simulink model "SchemaBlocFinala"  (R2024b)
settings: Solver=VariableStepAuto  StartTime=0.0  StopTime=1000  RelTol=1e-3
values from neighbouring files (symbols this model uses):
  A = 332.5    [date_indrumator.m]
  C = 9    [date_indrumator.m]
  h0 = 10.5    [date_indrumator.m]
  k = 0.035    [date_indrumator.m]    (also in proiect.m)
  k11 = k2^2 + 4*(k - k3)*k1    (= 0.08909684)    [date_indrumator.m]    (also in proiect.m = 0.08885985)
  k12 = 8*(k-k3)    (= 0.2848)    [date_indrumator.m]    (also in proiect.m)
  k13 = 2*(k-k3)    (= 0.0712)    [date_indrumator.m]    (also in proiect.m)
  k2 = -0.015    [date_indrumator.m]    (also in proiect.m = -0.0015)
  keta = 8*(10^-5)    (= 8e-05)    [date_indrumator.m]    (also in proiect.m)
  q0 = 29.18    [date_indrumator.m]
settings Model: Creator=Ruxandra  LastModifiedBy=Ruxandra

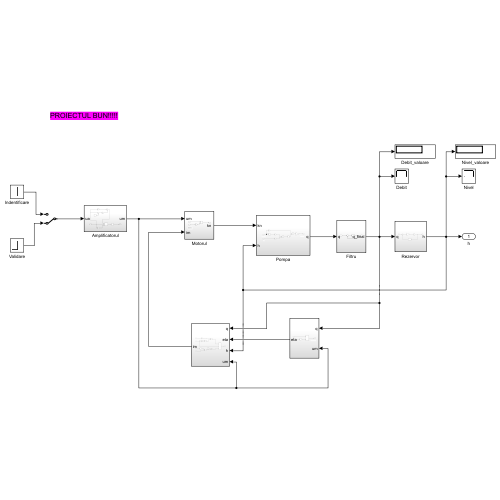
[thumbnail: Simulink's stored preview of the top-level diagram]
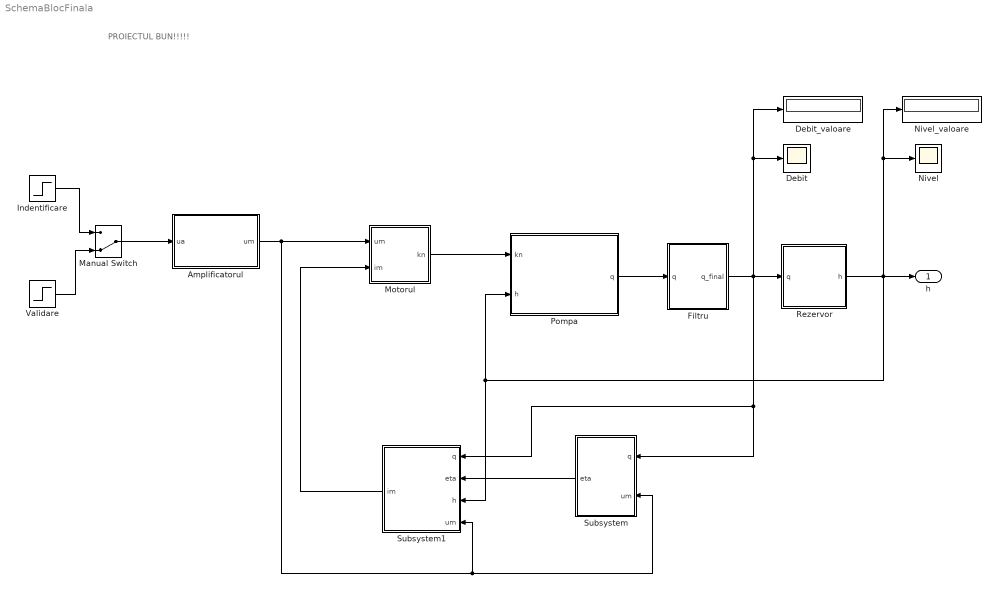
== system SchemaBlocFinala ==
  note: PROIECTUL BUN!!!!!
  Amplificatorul : Subsystem
  Debit : Scope
  Debit_valoare : Display
  Filtru : Subsystem
  Indentificare : Step  After=5  SampleTime=0
  Manual Switch : ManualSwitch  CurrentSetting=0
  Motorul : Subsystem
  Nivel : Scope
  Nivel_valoare : Display
  Pompa : Subsystem
  Rezervor : Subsystem
  Subsystem : Subsystem
  Subsystem1 : Subsystem
  Validare : Step  Before=5  After=5.5  SampleTime=0
  h : Outport
  wires:
  Motorul/1("kn ") -> Pompa/1(kn)
  Subsystem/1(eta) -> Subsystem1/2(eta)
  Subsystem1/1(im) -> Motorul/2(im)
  Pompa/1(q) -> Filtru/1(q)
  Filtru/1(q_final) -> Debit_valoare/1, Debit/1, Subsystem1/1(q), Subsystem/1(q), Rezervor/1(q)
  Rezervor/1(h) -> Pompa/2(h), Subsystem1/3(h), Nivel_valoare/1, Nivel/1, h/1
  Amplificatorul/1(um) -> Motorul/1(um), Subsystem1/4(um), Subsystem/2(um)
  Manual Switch/1 -> Amplificatorul/1(ua)
  Indentificare/1 -> Manual Switch/1
  Validare/1 -> Manual Switch/2

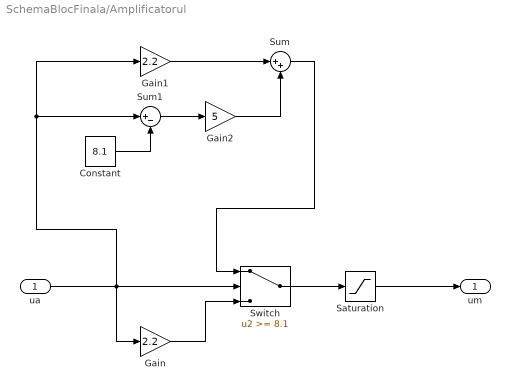
== system SchemaBlocFinala/Amplificatorul ==
  ua : Inport
  Constant : Constant  Value=8.1
  Gain : Gain  Gain=2.2
  Gain1 : Gain  Gain=2.2
  Gain2 : Gain  Gain=5
  Saturation : Saturate  UpperLimit=22  LowerLimit=0
  Sum : Sum  Inputs=|++
  Sum1 : Sum  Inputs=|+-
  Switch : Switch  Threshold=8.1  RndMeth=Nearest  SaturateOnIntegerOverflow=off  InputSameDT=off
  um : Outport
  wires:
  Gain/1 -> Switch/3
  Gain1/1 -> Sum/1
  Sum1/1 -> Gain2/1
  ua/1 -> Gain/1, Sum1/1, Gain1/1, Switch/2
  Saturation/1 -> um/1
  Constant/1 -> Sum1/2
  Sum/1 -> Switch/1
  Switch/1 -> Saturation/1
  Gain2/1 -> Sum/2

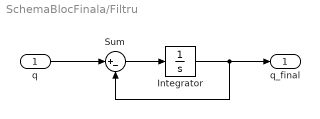
== system SchemaBlocFinala/Filtru ==
  q : Inport
  Integrator : Integrator  InitialCondition=q0
  Sum : Sum  Inputs=|+-
  q_final : Outport
  wires:
  Integrator/1 -> q_final/1, Sum/2
  q/1 -> Sum/1
  Sum/1 -> Integrator/1

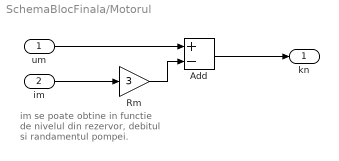
== system SchemaBlocFinala/Motorul ==
  note: im se poate obtine in functie de nivelul din rezervor, debitul si randamentul pompei.
  um : Inport
  im : Inport  Port=2
  Add : Sum  Inputs=+-
  Rm : Gain  Gain=3
  "kn " : Outport
  wires:
  Rm/1 -> Add/2
  Add/1 -> "kn "/1
  um/1 -> Add/1
  im/1 -> Rm/1

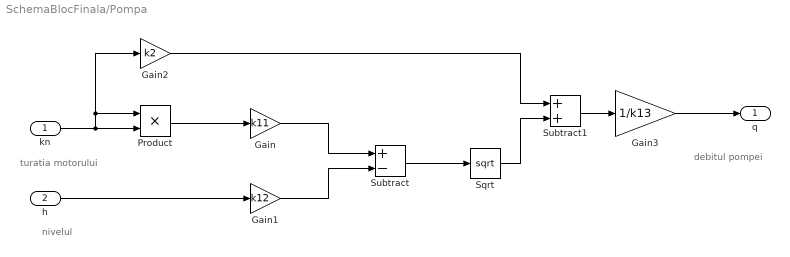
== system SchemaBlocFinala/Pompa ==
  note: nivelul
  note: turatia motorului
  note: debitul pompei
  kn : Inport
  h : Inport  Port=2
  Gain : Gain  Gain=k11
  Gain1 : Gain  Gain=k12
  Gain2 : Gain  Gain=k2
  Gain3 : Gain  Gain=1/k13
  Product : Product
  Sqrt : Sqrt
  Subtract : Sum  Inputs=+-
  Subtract1 : Sum
  q : Outport
  wires:
  Gain2/1 -> Subtract1/1
  kn/1 -> Product/1, Gain2/1, Product/2
  Gain3/1 -> q/1
  Product/1 -> Gain/1
  Gain1/1 -> Subtract/2
  Subtract/1 -> Sqrt/1
  h/1 -> Gain1/1
  Sqrt/1 -> Subtract1/2
  Gain/1 -> Subtract/1
  Subtract1/1 -> Gain3/1

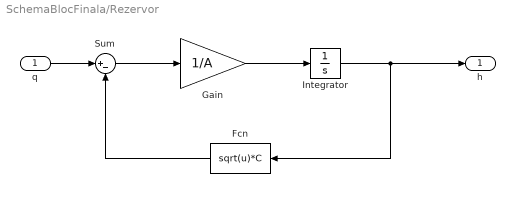
== system SchemaBlocFinala/Rezervor ==
  q : Inport
  Fcn : Fcn  Expr=sqrt(u)*C
  Gain : Gain  Gain=1/A
  Integrator : Integrator  InitialCondition=h0
  Sum : Sum  Inputs=|+-
  h : Outport
  wires:
  q/1 -> Sum/1
  Gain/1 -> Integrator/1
  Sum/1 -> Gain/1
  Integrator/1 -> Fcn/1, h/1
  Fcn/1 -> Sum/2

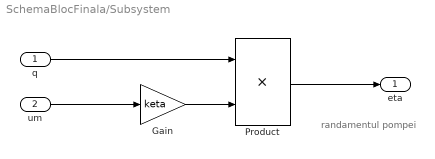
== system SchemaBlocFinala/Subsystem ==
  note: randamentul pompei
  q : Inport
  um : Inport  Port=2
  Gain : Gain  Gain=keta
  Product : Product
  eta : Outport
  wires:
  q/1 -> Product/1
  um/1 -> Gain/1
  Gain/1 -> Product/2
  Product/1 -> eta/1

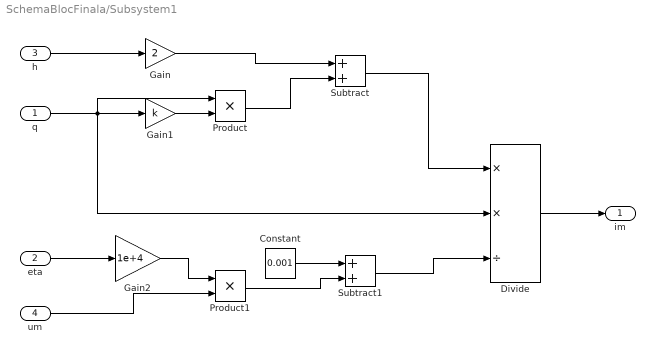
== system SchemaBlocFinala/Subsystem1 ==
  q : Inport
  eta : Inport  Port=2
  h : Inport  Port=3
  um : Inport  Port=4
  Constant : Constant  Value=0.001
  Divide : Product  Inputs=**/
  Gain : Gain  Gain=2
  Gain1 : Gain  Gain=k
  Gain2 : Gain  Gain=1e+4
  Product : Product
  Product1 : Product
  Subtract : Sum
  Subtract1 : Sum
  im : Outport
  wires:
  Subtract1/1 -> Divide/3
  Gain2/1 -> Product1/1
  h/1 -> Gain/1
  Subtract/1 -> Divide/1
  Product1/1 -> Subtract1/2
  eta/1 -> Gain2/1
  Gain1/1 -> Product/2
  um/1 -> Product1/2
  Constant/1 -> Subtract1/1
  Gain/1 -> Subtract/1
  Product/1 -> Subtract/2
  q/1 -> Divide/2, Gain1/1, Product/1
  Divide/1 -> im/1
